simulink model "Week1problem7"  (R2020b)
settings: Solver=VariableStepAuto  StartTime=0.0  StopTime=10.0  RelTol=1e-3
libraries: dspsrcs4 x1
settings Model: Creator=Admin  LastModifiedBy=Admin

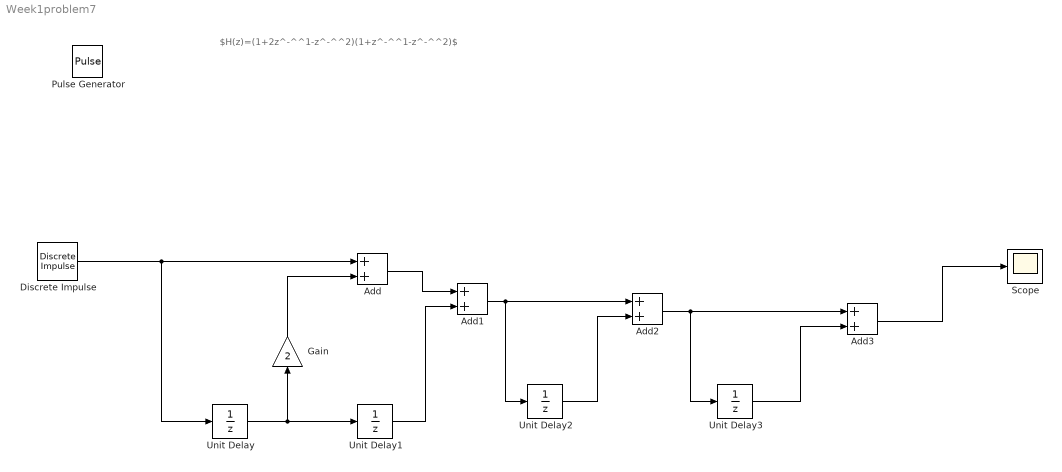
== system Week1problem7 ==
  note: $H(z)=(1+2z^-^^1-z^-^^2)(1+z^-^^1-z^-^^2)$
  Add{,1..3} (4 alike) : Sum
  Discrete Impulse : dspsrcs4/Discrete  Impulse  Delay=0  SampleTime=1  FrameSample=1  OutputFrames=off  dataType=double  isSigned=on  wordLen=16  udDataType=sfix(16)  fracBitsMode=Best precision  numFracBits=15  OutDataTypeStr=double  LastOutDataTypeStr=double
  Gain : Gain  Gain=2
  Pulse Generator : DiscretePulseGenerator  PulseType=Time based  Period=10  PulseWidth=5
  Scope : Scope
  Unit Delay{,1..3} (4 alike) : UnitDelay  SampleTime=-1  HasFrameUpgradeWarning=on
  wires:
  Discrete Impulse/1 -> Unit Delay/1, Add/1
  Add/1 -> Add1/1
  Unit Delay/1 -> Gain/1, Unit Delay1/1
  Gain/1 -> Add/2
  Unit Delay1/1 -> Add1/2
  Add1/1 -> Unit Delay2/1, Add2/1
  Unit Delay2/1 -> Add2/2
  Add2/1 -> Add3/1, Unit Delay3/1
  Unit Delay3/1 -> Add3/2
  Add3/1 -> Scope/1
